simulink model "Model_TranslationEngine64"  (R2022b)
settings: Solver=FixedStepDiscrete  StartTime=0.0  StopTime=5  RelTol=1e-3  EnableMultiTasking=on
InitFcn:
  | % Initialize model
  | ModelSettings=BTConfig.GetModelSettings();
  | 
  | ModelSettings.Validate();
  | 
  | ModelInit;
  | 
  | 
  | % load library data
  | GainLibrary_data;
  | % Load saved values from partition process
  | CapturedConstMask.LoadMapFromFile(bdroot)
StartFcn:
  | % make sure all the simulated RTC requests are found
  | %RTC_SIM_OBJ.ValidateREQs();
undefined symbols (not defined in the file or in its folder): AA, BPLP, Column, NumHFRefBPF, NumHFRefLPF, NumMusicChannels, Row, VolumeMuteConfig
libraries: TuneVar x925, TOP x490, FeaturePath x111, CapturedConstLib x52
(part 20 of 34)

== system Model_TranslationEngine64/ModelPreAmp/DecRate/Medusa5H1/SleepingBeauty/SleepingBeauty/Enabled/MuteControl ==
  MuteControl : Subsystem  mask(Blocklib MuteControl){Config=InnerLinkConfig, FeatureName=MuteControl}
      mask prompts: Config "MuteControlConfig"; FeatureName "Mask feature name:"
      mask help: This component is to be used in conjunction with 1 or more instances of the MuteRamper block. There is no mask for this component. It provides the control layer for Mute processing via an RTC and tune variable, muteControlRampTime.
      mask init: same as Model_TranslationEngine64/PostProcess/PostProcess/Mute/Mute/MuteControl
      mask Help: If this control block is being used in a "multi-instance" manner, i.e. it is contorlling two or more MuteRamper blocks, there is an additional step that must be done. The developer must add a function-triggered subsytem containing an AND logic gate, which will combine the notification completion signals of the multiple ramper instances. The output of this subsytem must then feed the NTF_done input of the MuteControl block.
      mask Callback Config: BTConfig.CallbackHideIfPresent(gcbh,{'FeatureName'});
      mask TypeOptions FeatureName: FeaturePath/FeatureName

== system Model_TranslationEngine64/ModelPreAmp/DecRate/Medusa5H1/SleepingBeauty/SleepingBeauty/Enabled/SleepingBeautyDR ==
  InnerLink : Subsystem  mask(Blocklib SleepingBeauty){Config=InnerLinkConfig, FeatureName=SleepingBeautyDR}
      mask prompts: Config "SleepingBeautyConfig"; FeatureName "Feature path name:"
      mask help:
      | This block is to be used in conjunction with the Balance block.
      |
      | For the Channel to Ramper Map, enter any of the following values:
      | 1 - left channel
      | 2 - right channel
      | 3 - center channel
      | 4 - mono channel
      | -1 - unused channel (will esentially be muted)
      | (For headrest speakers, choose a seat-centric ramper, i.e. Left Seat Left Ear and Left Seat Right Ear would both be considered "Left content", receiving a 1).
      |
      | Silent Extreme Mutes Bass: Check this box if the intention is for mono channels to be muted upon Silent Extreme
      |
      | If this block is being used in a multi-instance application, be sure to give independent names in each instance's mask.
      mask init:
      | blkh=gcbh;
      | Config=BTConfig.Assert(blkh,Config);
      | 
      | SleepingBeautyMask.Init(blkh);
      | 
      | % Set boundary conditions
      | rampRateBounds = [5,50000];
      | rampTimeBounds = [1,3000];
      | 
      | BTConfig.InitSetFeatureIfPresent(blkh,'FeatureName');
      | Config.Validate();
      mask Callback Config: BTConfig.CallbackHideIfPresent(gcbh,{'FeatureName'});
      mask TypeOptions FeatureName: FeaturePath/FeatureName

== system Model_TranslationEngine64/ModelPreAmp/DecRate/Medusa5H1/SleepingBeauty/SleepingBeauty/Enabled/SleepingBeautyFR ==
  InnerLink : Subsystem  mask(Blocklib SleepingBeauty){Config=InnerLinkConfig, FeatureName=SleepingBeautyFR}
      mask prompts: Config "SleepingBeautyConfig"; FeatureName "Feature path name:"
      mask help:
      | This block is to be used in conjunction with the Balance block.
      |
      | For the Channel to Ramper Map, enter any of the following values:
      | 1 - left channel
      | 2 - right channel
      | 3 - center channel
      | 4 - mono channel
      | -1 - unused channel (will esentially be muted)
      | (For headrest speakers, choose a seat-centric ramper, i.e. Left Seat Left Ear and Left Seat Right Ear would both be considered "Left content", receiving a 1).
      |
      | Silent Extreme Mutes Bass: Check this box if the intention is for mono channels to be muted upon Silent Extreme
      |
      | If this block is being used in a multi-instance application, be sure to give independent names in each instance's mask.
      mask init: same as Model_TranslationEngine64/ModelPreAmp/DecRate/Medusa5H1/SleepingBeauty/SleepingBeauty/Enabled/SleepingBeautyDR/InnerLink
      mask Callback Config: BTConfig.CallbackHideIfPresent(gcbh,{'FeatureName'});
      mask TypeOptions FeatureName: FeaturePath/FeatureName

== system Model_TranslationEngine64/ModelPreAmp/DecRate/Medusa5H1/VLS/Crosstalk Cancellation/Pooliir with Non-Trivial Translations/InnerLink ==
  PoolIirTunableWithReset : Subsystem  mask(Bose Pool IIR Tunable){FeatureName=IIR, Config=Config}
      mask prompts: FeatureName "Filter name/purpose"; Config "PoolIirTunableWithResetConfig"
      mask help:
      | Pool IIR Tunable is a configurable multi-channel IIR filter that supports one or more channels. This block offers flexibility of tuning the number of stages and coefficients. Different filter coefficients and number of stages (biquads) can be used for each channel filter. The Pool IIR Tunable block supports different implementations, which could be configured at build-time:
      |
      | (i)   Generic: IIR filter code not optimized for any processor
      | (ii)  SharcCore: IIR filters executing on core (uses pooliir.asm CRL)
      | (iii) SharcGulAccel: IIR filters executing on IIR hardware accelerator, offloading MIPS usage from core
      | (iv) SharcGxpAccel: IIR filters take advantage of additional accelerators available on GXP processor
      | (v)  Hexagon: TBD
      |
      | NOTE: When using Pool IIR for Sharc-plus based processors, the codeWorkMemory buffer and input buffer should always be mapped to L1 memory to optimize MIPS utilization and avoid audio artifacts.
      |
      | For more information, please see 'Help'.
      mask init:
      | blkh=gcbh;
      | Config=BTConfig.Assert(blkh,Config);
      | 
      | BTConfig.InitSetFeatureIfPresent(blkh,'FeatureName');
      | Config.Validate();
      | Config.DoMaskInit(blkh);
      mask Help:
      | <b>Input signals: </b>
      | AudioIn: input channels [frame size x number of channels]
      | ResetTrigger: trigger to reset internal state buffer (usually preferred as a post RMDL step)
      | 
      | <b>Output signals: </b>
      | AudioOut: output channels [frame size x number of channels]
      | 
      | <b>Mask parameters: </b>
      | PoolIirTunableWithResetConfig
      | Filter name/purpose
      mask TypeOptions FeatureName: FeaturePath/FeatureName
      mask Callback Config: BTConfig.CallbackHideIfPresent(gcbh,{'FeatureName'});
      mask Display: DrawPoolIirIcon;

== system Model_TranslationEngine64/ModelPreAmp/PreAmpPart1/NEARPreAmp/Monoizer/Monoizer/MonoizerStereo/MonoizerCalc ==
  TuneTOP1 : Subsystem  mask(Talaria Trivial Tune TOP){TriggerInit=[385 412 535 498], TopName=G, TuneName=G, DataTypeOut=single, MaskValue=Config.G, TunabilityNumber=1, MinValue=[], MaxValue=[], BankNumber=0, PreOverlay=false, PostOverlay=false, UseSameName=on}
      mask prompts: TriggerInit "Hidden: MoveFcn redraw"; TopName "Name:"; TuneName "Name of TuneVar:"; DataTypeOut "Data type:"; MaskValue "Default Value:"; TunabilityNumber "Tunability:"; MinValue "Min Value:"; MaxValue "Max Value:"; BankNumber "Target memory bank number:"; PreOverlay "Requires pre-overlay action:"; PostOverlay "Requires post-overlay action:"; UseSameName "Use same name for tune variable and TOP"
      mask help: The TuneTOP block encapsultes a Target Overlay Parameter, a Tune Variable, and a Trivial Translation between them.
      mask init:
      | [ok,activeTopPath,activeTunePath] = TuneTOP_Mask.Init(gcbh);
      settings: MoveFcn=TuneTOP_Mask.CB_TriggerInit(gcbh);
      mask Callback TriggerInit: TuneTOP_Mask.CB_TriggerInit(gcbh);
      mask TypeOptions TopName: TOP/TopName
      mask TypeOptions TuneName: Tune Variable/TuneName
      mask TypeOptions DataTypeOut: TOP/DataTypeOut
      mask TypeOptions MaskValue: Tune Variable/MaskValue
      mask TypeOptions TunabilityNumber: Tune Variable/TunabilityNumber
      mask Callback TunabilityNumber: TuneVarMask.CB_TunabilityNumber(gcbh);
      mask TypeOptions MinValue: Tune Variable/MinValue
      mask TypeOptions MaxValue: Tune Variable/MaxValue
      mask TypeOptions BankNumber: TOP/BankNumber
      mask TypeOptions PreOverlay: TOP/PreOverlay
      mask TypeOptions PostOverlay: TOP/PostOverlay
      mask Callback UseSameName: TuneTOP_Mask.CB_UseSameName(gcbh);
      mask DialogControl toolPanel Prompt: Tuning Tool Hints
      mask DialogControl DescriptionGroup Prompt: Description
      mask DialogControl EditDescription Prompt: Edit Description
      mask DialogControl EditDescription Callback: TuneTOP_Mask.CB_EditDescription(gcbh);
      mask DialogControl TunabilityText Prompt: Easy: Changes nearly every tuning.
      mask DialogControl AdvancedPanel Prompt: Advanced
      mask DialogControl ConvertToFullTranslation Prompt: Irreversible conversion to full translation
      mask DialogControl ConvertToFullTranslation Callback: TuneTOP_Mask.CB_ConvertToFullTranslation(gcbh);
      mask DialogControl ErrorContainer Prompt: Error Messages
      mask Display:
      | % retrieve icon definition
      | [path,w,h] = TuneTOP_Mask.Icon();
      | 
      | % retrieve the block's pixel size
      | pos = get(gcbh,'position');
      | bw = pos(3) - pos(1);
      | bh = pos(4) - pos(2);
      | 
      | % draw centered icon
      | xAdj = bw/2 - w/2 + 5;
      | yAdj = bh/2 - h/2 + 4;
      | for i=1:length(path)
      | 	patch(path(i).x+xAdj, path(i).y+yAdj, path(i).rgb);
      | end
      | 
      | % show the top name or an X
      | if (exist('ok','var') && ok)
      | 	text(bw*0.5, bh*0.2, activeTopPath, 'horizontalAlignment', 'center');
      | 	patch(0,0,[1 1 1]);
      | 	patch(bw,bh,[1 1 1]);
      | else
      | 	tx=bw*0.03;
      | 	ty=bh*0.03;
      | 	patch([0 tx bw bw-tx], [ty 0 bh-ty bh], [1 0 0]);
      | 	patch([0 bw-tx bw tx], [bh-ty 0 ty bh], [1 0 0]);
      | end

== system Model_TranslationEngine64/NEAR/Near1p1/FrProc/Subsystem/FsEQFr/Pooliir/PoolIirTunableWithReset ==
  CapturedTuneConst : CapturedConstLib/CapturedConst  TriggerInit=[-600 302 -500 338]  Role=Automatic
      settings: SourceProductName=Bose Talaria
  FeaturePath : FeaturePath/FeaturePath  FeatureName=Pooliir  IsGroup=off  GroupNumber=-1  IsModule=off  TriggerInit=[-750 -81 -635 26]
      settings: SourceProductName=Bose Talaria
  TOP : TOP/TOP  TriggerInit=[-145 187 5 243]  TopName=PooliirNumStages  DataTypeOut=uint32  BankNumber=0  PreOverlay=false  PostOverlay=Config.VariantObj.PostOverlayRequired  Role=Automatic
      settings: SourceProductName=Bose Talaria
  TOP1 : TOP/TOP  TriggerInit=[-140 277 10 333]  TopName=pooliirCoeffs  DataTypeOut=single  BankNumber=0  PreOverlay=false  PostOverlay=Config.VariantObj.PostOverlayRequired  Role=Automatic
      settings: SourceProductName=Bose Talaria
  TranslateTrigger : TuneVar/TranslateTrigger  TriggerInit=[-339 35 -301 90]
      settings: SourceProductName=Bose Talaria
  Translation : MATLAB Function  TreatAsAtomicUnit=on  mask{MaxNumStages=Config.MaxNumStages, VariantUint8=Config.Variant.Uint8Str}
      mask prompts: VariantUint8 "Variant"
  Tune Variable1 : TuneVar/TuneVar  TuneName=numStages  SpecifyMaxSize=off  VariableDim=1 (Row)  MaxSize=[1 1]  TunabilityNumber=1  MinValue=[]  MaxValue=[]  TriggerInit=[-750 235 -580 285]  MaskValue=Config.TuneDefaults.NumStages
      settings: SourceProductName=Bose Talaria
  Tune Variable2 : TuneVar/TuneVar  TuneName=sosCoefficients  SpecifyMaxSize=on  VariableDim=1 (Row)  MaxSize=[Config.MaxNumStages 6]  TunabilityNumber=1  MinValue=[]  MaxValue=[]  TriggerInit=[-750 175 -580 225]  MaskValue=Config.TuneDefaults.SosCoefficients
      settings: SourceProductName=Bose Talaria
  wires:
  TranslateTrigger/1 -> Translation/Trigger
  Tune Variable2/1 -> Translation/1(RawSOS)  "sosCoefficients"
  Translation/2(PoolCoeffs) -> TOP1/1
  Translation/1(PoolNumStages) -> TOP/1
  Tune Variable1/1 -> Translation/2(NumStages)  "numStages"
  CapturedTuneConst/1 -> Translation/3(NumChannels)

== system Model_TranslationEngine64/NEAR/Near1p1/FrProc/Subsystem/FsEQFr/Subsystem1/Subsystem ==
  Tune Variable : TuneVar/TuneVar  TuneName=f1_del  SpecifyMaxSize=off  VariableDim=1 (Row)  MaxSize=[1 1]  TunabilityNumber=1  MinValue=[]  MaxValue=[]  TriggerInit=[20 20 190 70]  MaskValue=Config.f1_del
      settings: SourceProductName=Bose Talaria
  Tune Variable1 : TuneVar/TuneVar  TuneName=f2_del  SpecifyMaxSize=off  VariableDim=1 (Row)  MaxSize=[1 1]  TunabilityNumber=1  MinValue=[]  MaxValue=[]  TriggerInit=[20 155 190 205]  MaskValue=Config.f2_del
      settings: SourceProductName=Bose Talaria
  Tune Variable2 : TuneVar/TuneVar  TuneName=f3_del  SpecifyMaxSize=off  VariableDim=1 (Row)  MaxSize=[1 1]  TunabilityNumber=1  MinValue=[]  MaxValue=[]  TriggerInit=[20 290 190 340]  MaskValue=Config.f3_del
      settings: SourceProductName=Bose Talaria
  Tune Variable3 : TuneVar/TuneVar  TuneName=f4_del  SpecifyMaxSize=off  VariableDim=1 (Row)  MaxSize=[1 1]  TunabilityNumber=1  MinValue=[]  MaxValue=[]  TriggerInit=[20 425 190 475]  MaskValue=Config.f4_del
      settings: SourceProductName=Bose Talaria
  Tune Variable4 : TuneVar/TuneVar  TuneName=f5_del  SpecifyMaxSize=off  VariableDim=1 (Row)  MaxSize=[1 1]  TunabilityNumber=1  MinValue=[]  MaxValue=[]  TriggerInit=[20 560 190 610]  MaskValue=Config.f5_del
      settings: SourceProductName=Bose Talaria
  Tune Variable5 : TuneVar/TuneVar  TuneName=f6_del  SpecifyMaxSize=off  VariableDim=1 (Row)  MaxSize=[1 1]  TunabilityNumber=1  MinValue=[]  MaxValue=[]  TriggerInit=[20 695 190 745]  MaskValue=Config.f6_del
      settings: SourceProductName=Bose Talaria
  Tune Variable7 : TuneVar/TuneVar  TuneName=f7_del  SpecifyMaxSize=off  VariableDim=1 (Row)  MaxSize=[1 1]  TunabilityNumber=1  MinValue=[]  MaxValue=[]  TriggerInit=[20 825 190 875]  MaskValue=Config.f7_del
      settings: SourceProductName=Bose Talaria
  f1 : Outport
  f2 : Outport  Port=2
  f3 : Outport  Port=3
  f4 : Outport  Port=4
  f5 : Outport  Port=5
  f6 : Outport  Port=6
  f7 : Outport  Port=7
  wires:
  Tune Variable5/1 -> f6/1  "f6_del"
  Tune Variable2/1 -> f3/1  "f3_del"
  Tune Variable7/1 -> f7/1  "f7_del"
  Tune Variable/1 -> f1/1  "f1_del"
  Tune Variable1/1 -> f2/1  "f2_del"
  Tune Variable3/1 -> f4/1  "f4_del"
  Tune Variable4/1 -> f5/1  "f5_del"

== system Model_TranslationEngine64/NEAR/Near1p1/FrProc/Subsystem/HrEQFr/PoolIirTunable/PoolIirTunableWithReset ==
  CapturedTuneConst : CapturedConstLib/CapturedConst  TriggerInit=[-600 302 -500 338]  Role=Automatic
      settings: SourceProductName=Bose Talaria
  FeaturePath : FeaturePath/FeaturePath  FeatureName=PoolIirTunable  IsGroup=off  GroupNumber=-1  IsModule=off  TriggerInit=[-750 -81 -635 26]
      settings: SourceProductName=Bose Talaria
  TOP : TOP/TOP  TriggerInit=[-145 187 5 243]  TopName=PooliirNumStages  DataTypeOut=uint32  BankNumber=0  PreOverlay=false  PostOverlay=Config.VariantObj.PostOverlayRequired  Role=Automatic
      settings: SourceProductName=Bose Talaria
  TOP1 : TOP/TOP  TriggerInit=[-140 277 10 333]  TopName=pooliirCoeffs  DataTypeOut=single  BankNumber=0  PreOverlay=false  PostOverlay=Config.VariantObj.PostOverlayRequired  Role=Automatic
      settings: SourceProductName=Bose Talaria
  TranslateTrigger : TuneVar/TranslateTrigger  TriggerInit=[-339 35 -301 90]
      settings: SourceProductName=Bose Talaria
  Translation : MATLAB Function  TreatAsAtomicUnit=on  mask{MaxNumStages=Config.MaxNumStages, VariantUint8=Config.Variant.Uint8Str}
      mask prompts: VariantUint8 "Variant"
  Tune Variable1 : TuneVar/TuneVar  TuneName=numStages  SpecifyMaxSize=off  VariableDim=1 (Row)  MaxSize=[1 1]  TunabilityNumber=1  MinValue=[]  MaxValue=[]  TriggerInit=[-750 235 -580 285]  MaskValue=Config.TuneDefaults.NumStages
      settings: SourceProductName=Bose Talaria
  Tune Variable2 : TuneVar/TuneVar  TuneName=sosCoefficients  SpecifyMaxSize=on  VariableDim=1 (Row)  MaxSize=[Config.MaxNumStages 6]  TunabilityNumber=1  MinValue=[]  MaxValue=[]  TriggerInit=[-750 175 -580 225]  MaskValue=Config.TuneDefaults.SosCoefficients
      settings: SourceProductName=Bose Talaria
  wires:
  TranslateTrigger/1 -> Translation/Trigger
  Tune Variable2/1 -> Translation/1(RawSOS)  "sosCoefficients"
  Translation/2(PoolCoeffs) -> TOP1/1
  Translation/1(PoolNumStages) -> TOP/1
  Tune Variable1/1 -> Translation/2(NumStages)  "numStages"
  CapturedTuneConst/1 -> Translation/3(NumChannels)

== system Model_TranslationEngine64/NEAR/Near1p1/FrProc/Subsystem/HrEQFr/Subsystem2/Subsystem ==
  Tune Variable1 : TuneVar/TuneVar  TuneName=driver_src1  SpecifyMaxSize=off  VariableDim=1 (Row)  MaxSize=[1 1]  TunabilityNumber=1  MinValue=[]  MaxValue=[]  TriggerInit=[35 385 205 435]  MaskValue=Config.driver_src1
      settings: SourceProductName=Bose Talaria
  Tune Variable2 : TuneVar/TuneVar  TuneName=driver_src2  SpecifyMaxSize=off  VariableDim=1 (Row)  MaxSize=[1 1]  TunabilityNumber=1  MinValue=[]  MaxValue=[]  TriggerInit=[35 515 205 565]  MaskValue=Config.driver_src2
      settings: SourceProductName=Bose Talaria
  Tune Variable3 : TuneVar/TuneVar  TuneName=driver_src3  SpecifyMaxSize=off  VariableDim=1 (Row)  MaxSize=[1 1]  TunabilityNumber=1  MinValue=[]  MaxValue=[]  TriggerInit=[35 620 205 670]  MaskValue=Config.driver_src3
      settings: SourceProductName=Bose Talaria
  Tune Variable4 : TuneVar/TuneVar  TuneName=driver_src4  SpecifyMaxSize=off  VariableDim=1 (Row)  MaxSize=[1 1]  TunabilityNumber=1  MinValue=[]  MaxValue=[]  TriggerInit=[35 750 205 800]  MaskValue=Config.driver_src4
      settings: SourceProductName=Bose Talaria
  Tune Variable5 : TuneVar/TuneVar  TuneName=passenger_src1  SpecifyMaxSize=off  VariableDim=1 (Row)  MaxSize=[1 1]  TunabilityNumber=1  MinValue=[]  MaxValue=[]  TriggerInit=[35 880 205 930]  MaskValue=Config.passenger_src1
      settings: SourceProductName=Bose Talaria
  Tune Variable6 : TuneVar/TuneVar  TuneName=passenger_src3  SpecifyMaxSize=off  VariableDim=1 (Row)  MaxSize=[1 1]  TunabilityNumber=1  MinValue=[]  MaxValue=[]  TriggerInit=[35 1140 205 1190]  MaskValue=Config.passenger_src3
      settings: SourceProductName=Bose Talaria
  Tune Variable7 : TuneVar/TuneVar  TuneName=passenger_src2  SpecifyMaxSize=off  VariableDim=1 (Row)  MaxSize=[1 1]  TunabilityNumber=1  MinValue=[]  MaxValue=[]  TriggerInit=[35 1010 205 1060]  MaskValue=Config.passenger_src2
      settings: SourceProductName=Bose Talaria
  Tune Variable8 : TuneVar/TuneVar  TuneName=passenger_src4  SpecifyMaxSize=off  VariableDim=1 (Row)  MaxSize=[1 1]  TunabilityNumber=1  MinValue=[]  MaxValue=[]  TriggerInit=[30 1285 200 1335]  MaskValue=Config.passenger_src4
      settings: SourceProductName=Bose Talaria
  driver_src1 : Outport
  driver_src2 : Outport  Port=2
  driver_src3 : Outport  Port=3
  driver_src4 : Outport  Port=4
  passenger_src1 : Outport  Port=5
  passenger_src2 : Outport  Port=6
  passenger_src3 : Outport  Port=7
  passenger_src4 : Outport  Port=8
  wires:
  Tune Variable5/1 -> passenger_src1/1  "passenger_src1"
  Tune Variable7/1 -> passenger_src2/1  "passenger_src2"
  Tune Variable8/1 -> passenger_src4/1  "passenger_src4"
  Tune Variable6/1 -> passenger_src3/1  "passenger_src3"
  Tune Variable4/1 -> driver_src4/1  "driver_src4"
  Tune Variable3/1 -> driver_src3/1  "driver_src3"
  Tune Variable2/1 -> driver_src2/1  "driver_src2"
  Tune Variable1/1 -> driver_src1/1  "driver_src1"

== system Model_TranslationEngine64/NEAR/Near1p1/FrProc/Subsystem/Upmixer1p1Fr/Subsystem1/Subsystem ==
  Tune Variable : TuneVar/TuneVar  TuneName=f1_mix  SpecifyMaxSize=off  VariableDim=1 (Row)  MaxSize=[1 1]  TunabilityNumber=1  MinValue=[]  MaxValue=[]  TriggerInit=[20 20 190 70]  MaskValue=Config.TuneDefaults.f1_mix
      settings: SourceProductName=Bose Talaria
  Tune Variable1 : TuneVar/TuneVar  TuneName=f2_mix  SpecifyMaxSize=off  VariableDim=1 (Row)  MaxSize=[1 1]  TunabilityNumber=1  MinValue=[]  MaxValue=[]  TriggerInit=[20 155 190 205]  MaskValue=Config.TuneDefaults.f2_mix
      settings: SourceProductName=Bose Talaria
  Tune Variable2 : TuneVar/TuneVar  TuneName=f3_mix  SpecifyMaxSize=off  VariableDim=1 (Row)  MaxSize=[1 1]  TunabilityNumber=1  MinValue=[]  MaxValue=[]  TriggerInit=[20 290 190 340]  MaskValue=Config.TuneDefaults.f3_mix
      settings: SourceProductName=Bose Talaria
  Tune Variable3 : TuneVar/TuneVar  TuneName=f4_mix  SpecifyMaxSize=off  VariableDim=1 (Row)  MaxSize=[1 1]  TunabilityNumber=1  MinValue=[]  MaxValue=[]  TriggerInit=[20 425 190 475]  MaskValue=Config.TuneDefaults.f4_mix
      settings: SourceProductName=Bose Talaria
  Tune Variable4 : TuneVar/TuneVar  TuneName=f5_mix  SpecifyMaxSize=off  VariableDim=1 (Row)  MaxSize=[1 1]  TunabilityNumber=1  MinValue=[]  MaxValue=[]  TriggerInit=[20 560 190 610]  MaskValue=Config.TuneDefaults.f5_mix
      settings: SourceProductName=Bose Talaria
  Tune Variable5 : TuneVar/TuneVar  TuneName=f6_mix  SpecifyMaxSize=off  VariableDim=1 (Row)  MaxSize=[1 1]  TunabilityNumber=1  MinValue=[]  MaxValue=[]  TriggerInit=[20 695 190 745]  MaskValue=Config.TuneDefaults.f6_mix
      settings: SourceProductName=Bose Talaria
  Tune Variable7 : TuneVar/TuneVar  TuneName=f7_mix  SpecifyMaxSize=off  VariableDim=1 (Row)  MaxSize=[1 1]  TunabilityNumber=1  MinValue=[]  MaxValue=[]  TriggerInit=[20 825 190 875]  MaskValue=Config.TuneDefaults.f7_mix
      settings: SourceProductName=Bose Talaria
  f1 : Outport
  f2 : Outport  Port=2
  f3 : Outport  Port=3
  f4 : Outport  Port=4
  f5 : Outport  Port=5
  f6 : Outport  Port=6
  f7 : Outport  Port=7
  wires:
  Tune Variable5/1 -> f6/1  "f6_mix"
  Tune Variable2/1 -> f3/1  "f3_mix"
  Tune Variable7/1 -> f7/1  "f7_mix"
  Tune Variable/1 -> f1/1  "f1_mix"
  Tune Variable1/1 -> f2/1  "f2_mix"
  Tune Variable3/1 -> f4/1  "f4_mix"
  Tune Variable4/1 -> f5/1  "f5_mix"

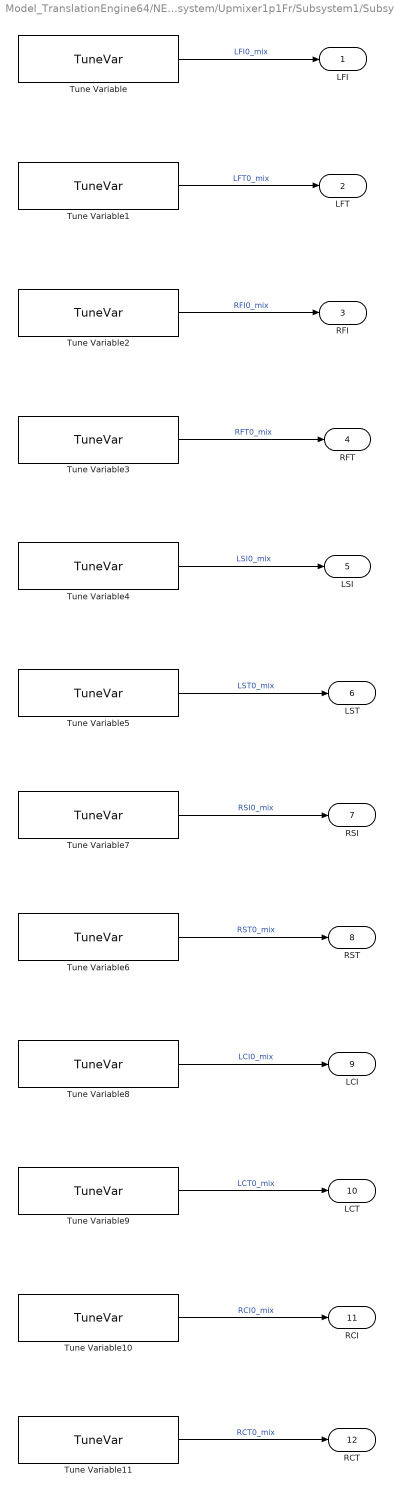
== system Model_TranslationEngine64/NEAR/Near1p1/FrProc/Subsystem/Upmixer1p1Fr/Subsystem1/Subsystem1 ==
  Tune Variable : TuneVar/TuneVar  TuneName=LFI0_mix  SpecifyMaxSize=off  VariableDim=1 (Row)  MaxSize=[1 1]  TunabilityNumber=1  MinValue=[]  MaxValue=[]  TriggerInit=[1315 -1070 1485 -1020]  MaskValue=Config.TuneDefaults.LFI0_mix
      settings: SourceProductName=Bose Talaria
  Tune Variable1 : TuneVar/TuneVar  TuneName=LFT0_mix  SpecifyMaxSize=off  VariableDim=1 (Row)  MaxSize=[1 1]  TunabilityNumber=1  MinValue=[]  MaxValue=[]  TriggerInit=[1315 -935 1485 -885]  MaskValue=Config.TuneDefaults.LFT0_mix
      settings: SourceProductName=Bose Talaria
  Tune Variable10 : TuneVar/TuneVar  TuneName=RCI0_mix  SpecifyMaxSize=off  VariableDim=1 (Row)  MaxSize=[1 1]  TunabilityNumber=1  MinValue=[]  MaxValue=[]  TriggerInit=[1315 270 1485 320]  MaskValue=Config.TuneDefaults.RCI0_mix
      settings: SourceProductName=Bose Talaria
  Tune Variable11 : TuneVar/TuneVar  TuneName=RCT0_mix  SpecifyMaxSize=off  VariableDim=1 (Row)  MaxSize=[1 1]  TunabilityNumber=1  MinValue=[]  MaxValue=[]  TriggerInit=[1315 400 1485 450]  MaskValue=Config.TuneDefaults.RCT0_mix
      settings: SourceProductName=Bose Talaria
  Tune Variable2 : TuneVar/TuneVar  TuneName=RFI0_mix  SpecifyMaxSize=off  VariableDim=1 (Row)  MaxSize=[1 1]  TunabilityNumber=1  MinValue=[]  MaxValue=[]  TriggerInit=[1315 -800 1485 -750]  MaskValue=Config.TuneDefaults.RFI0_mix
      settings: SourceProductName=Bose Talaria
  Tune Variable3 : TuneVar/TuneVar  TuneName=RFT0_mix  SpecifyMaxSize=off  VariableDim=1 (Row)  MaxSize=[1 1]  TunabilityNumber=1  MinValue=[]  MaxValue=[]  TriggerInit=[1315 -665 1485 -615]  MaskValue=Config.TuneDefaults.RFT0_mix
      settings: SourceProductName=Bose Talaria
  Tune Variable4 : TuneVar/TuneVar  TuneName=LSI0_mix  SpecifyMaxSize=off  VariableDim=1 (Row)  MaxSize=[1 1]  TunabilityNumber=1  MinValue=[]  MaxValue=[]  TriggerInit=[1315 -530 1485 -480]  MaskValue=Config.TuneDefaults.LSI0_mix
      settings: SourceProductName=Bose Talaria
  Tune Variable5 : TuneVar/TuneVar  TuneName=LST0_mix  SpecifyMaxSize=off  VariableDim=1 (Row)  MaxSize=[1 1]  TunabilityNumber=1  MinValue=[]  MaxValue=[]  TriggerInit=[1315 -395 1485 -345]  MaskValue=Config.TuneDefaults.LST0_mix
      settings: SourceProductName=Bose Talaria
  Tune Variable6 : TuneVar/TuneVar  TuneName=RST0_mix  SpecifyMaxSize=off  VariableDim=1 (Row)  MaxSize=[1 1]  TunabilityNumber=1  MinValue=[]  MaxValue=[]  TriggerInit=[1315 -135 1485 -85]  MaskValue=Config.TuneDefaults.RST0_mix
      settings: SourceProductName=Bose Talaria
  Tune Variable7 : TuneVar/TuneVar  TuneName=RSI0_mix  SpecifyMaxSize=off  VariableDim=1 (Row)  MaxSize=[1 1]  TunabilityNumber=1  MinValue=[]  MaxValue=[]  TriggerInit=[1315 -265 1485 -215]  MaskValue=Config.TuneDefaults.RSI0_mix
      settings: SourceProductName=Bose Talaria
  Tune Variable8 : TuneVar/TuneVar  TuneName=LCI0_mix  SpecifyMaxSize=off  VariableDim=1 (Row)  MaxSize=[1 1]  TunabilityNumber=1  MinValue=[]  MaxValue=[]  TriggerInit=[20 1090 190 1140]  MaskValue=Config.TuneDefaults.LCI0_mix
      settings: SourceProductName=Bose Talaria
  Tune Variable9 : TuneVar/TuneVar  TuneName=LCT0_mix  SpecifyMaxSize=off  VariableDim=1 (Row)  MaxSize=[1 1]  TunabilityNumber=1  MinValue=[]  MaxValue=[]  TriggerInit=[1315 135 1485 185]  MaskValue=Config.TuneDefaults.LCT0_mix
      settings: SourceProductName=Bose Talaria
  LFI : Outport
  LFT : Outport  Port=2
  RFI : Outport  Port=3
  RFT : Outport  Port=4
  LSI : Outport  Port=5
  LST : Outport  Port=6
  RSI : Outport  Port=7
  RST : Outport  Port=8
  LCI : Outport  Port=9
  LCT : Outport  Port=10
  RCI : Outport  Port=11
  RCT : Outport  Port=12
  wires:
  Tune Variable1/1 -> LFT/1  "LFT0_mix"
  Tune Variable11/1 -> RCT/1  "RCT0_mix"
  Tune Variable6/1 -> RST/1  "RST0_mix"
  Tune Variable3/1 -> RFT/1  "RFT0_mix"
  Tune Variable/1 -> LFI/1  "LFI0_mix"
  Tune Variable2/1 -> RFI/1  "RFI0_mix"
  Tune Variable7/1 -> RSI/1  "RSI0_mix"
  Tune Variable4/1 -> LSI/1  "LSI0_mix"
  Tune Variable8/1 -> LCI/1  "LCI0_mix"
  Tune Variable5/1 -> LST/1  "LST0_mix"
  Tune Variable9/1 -> LCT/1  "LCT0_mix"
  Tune Variable10/1 -> RCI/1  "RCI0_mix"

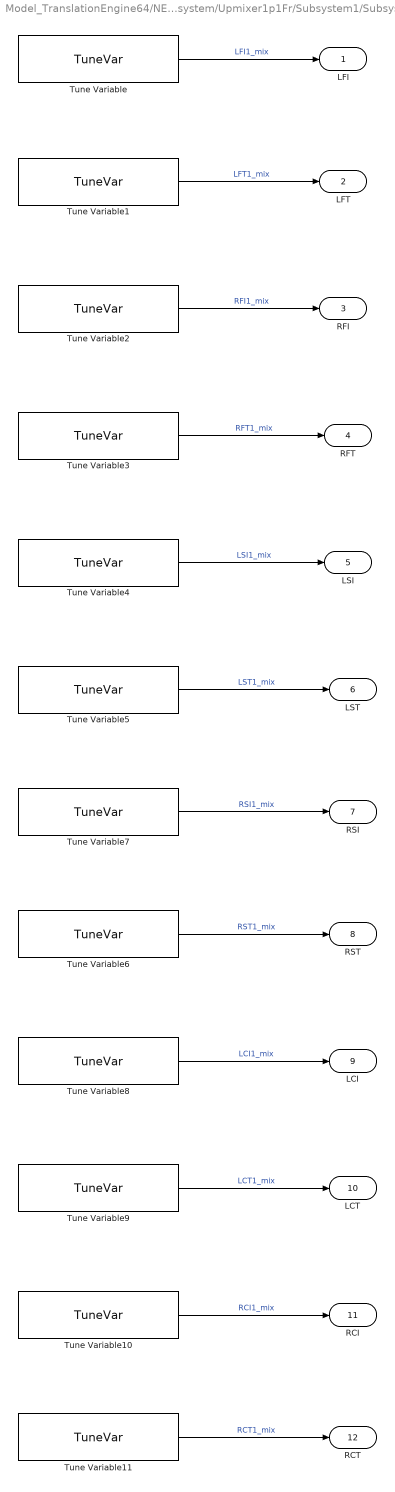
== system Model_TranslationEngine64/NEAR/Near1p1/FrProc/Subsystem/Upmixer1p1Fr/Subsystem1/Subsystem2 ==
  Tune Variable : TuneVar/TuneVar  TuneName=LFI1_mix  SpecifyMaxSize=off  VariableDim=1 (Row)  MaxSize=[1 1]  TunabilityNumber=1  MinValue=[]  MaxValue=[]  TriggerInit=[1315 910 1485 960]  MaskValue=Config.TuneDefaults.LFI1_mix
      settings: SourceProductName=Bose Talaria
  Tune Variable1 : TuneVar/TuneVar  TuneName=LFT1_mix  SpecifyMaxSize=off  VariableDim=1 (Row)  MaxSize=[1 1]  TunabilityNumber=1  MinValue=[]  MaxValue=[]  TriggerInit=[1315 1040 1485 1090]  MaskValue=Config.TuneDefaults.LFT1_mix
      settings: SourceProductName=Bose Talaria
  Tune Variable10 : TuneVar/TuneVar  TuneName=RCI1_mix  SpecifyMaxSize=off  VariableDim=1 (Row)  MaxSize=[1 1]  TunabilityNumber=1  MinValue=[]  MaxValue=[]  TriggerInit=[1315 2245 1485 2295]  MaskValue=Config.TuneDefaults.RCI1_mix
      settings: SourceProductName=Bose Talaria
  Tune Variable11 : TuneVar/TuneVar  TuneName=RCT1_mix  SpecifyMaxSize=off  VariableDim=1 (Row)  MaxSize=[1 1]  TunabilityNumber=1  MinValue=[]  MaxValue=[]  TriggerInit=[1315 2375 1485 2425]  MaskValue=Config.TuneDefaults.RCT1_mix
      settings: SourceProductName=Bose Talaria
  Tune Variable2 : TuneVar/TuneVar  TuneName=RFI1_mix  SpecifyMaxSize=off  VariableDim=1 (Row)  MaxSize=[1 1]  TunabilityNumber=1  MinValue=[]  MaxValue=[]  TriggerInit=[1315 1175 1485 1225]  MaskValue=Config.TuneDefaults.RFI1_mix
      settings: SourceProductName=Bose Talaria
  Tune Variable3 : TuneVar/TuneVar  TuneName=RFT1_mix  SpecifyMaxSize=off  VariableDim=1 (Row)  MaxSize=[1 1]  TunabilityNumber=1  MinValue=[]  MaxValue=[]  TriggerInit=[1315 1310 1485 1360]  MaskValue=Config.TuneDefaults.RFT1_mix
      settings: SourceProductName=Bose Talaria
  Tune Variable4 : TuneVar/TuneVar  TuneName=LSI1_mix  SpecifyMaxSize=off  VariableDim=1 (Row)  MaxSize=[1 1]  TunabilityNumber=1  MinValue=[]  MaxValue=[]  TriggerInit=[1315 1445 1485 1495]  MaskValue=Config.TuneDefaults.LSI1_mix
      settings: SourceProductName=Bose Talaria
  Tune Variable5 : TuneVar/TuneVar  TuneName=LST1_mix  SpecifyMaxSize=off  VariableDim=1 (Row)  MaxSize=[1 1]  TunabilityNumber=1  MinValue=[]  MaxValue=[]  TriggerInit=[1315 1580 1485 1630]  MaskValue=Config.TuneDefaults.LST1_mix
      settings: SourceProductName=Bose Talaria
  Tune Variable6 : TuneVar/TuneVar  TuneName=RST1_mix  SpecifyMaxSize=off  VariableDim=1 (Row)  MaxSize=[1 1]  TunabilityNumber=1  MinValue=[]  MaxValue=[]  TriggerInit=[1315 1840 1485 1890]  MaskValue=Config.TuneDefaults.RST1_mix
      settings: SourceProductName=Bose Talaria
  Tune Variable7 : TuneVar/TuneVar  TuneName=RSI1_mix  SpecifyMaxSize=off  VariableDim=1 (Row)  MaxSize=[1 1]  TunabilityNumber=1  MinValue=[]  MaxValue=[]  TriggerInit=[1315 1710 1485 1760]  MaskValue=Config.TuneDefaults.RSI1_mix
      settings: SourceProductName=Bose Talaria
  Tune Variable8 : TuneVar/TuneVar  TuneName=LCI1_mix  SpecifyMaxSize=off  VariableDim=1 (Row)  MaxSize=[1 1]  TunabilityNumber=1  MinValue=[]  MaxValue=[]  TriggerInit=[1315 1975 1485 2025]  MaskValue=Config.TuneDefaults.LCI1_mix
      settings: SourceProductName=Bose Talaria
  Tune Variable9 : TuneVar/TuneVar  TuneName=LCT1_mix  SpecifyMaxSize=off  VariableDim=1 (Row)  MaxSize=[1 1]  TunabilityNumber=1  MinValue=[]  MaxValue=[]  TriggerInit=[1315 2110 1485 2160]  MaskValue=Config.TuneDefaults.LCT1_mix
      settings: SourceProductName=Bose Talaria
  LFI : Outport
  LFT : Outport  Port=2
  RFI : Outport  Port=3
  RFT : Outport  Port=4
  LSI : Outport  Port=5
  LST : Outport  Port=6
  RSI : Outport  Port=7
  RST : Outport  Port=8
  LCI : Outport  Port=9
  LCT : Outport  Port=10
  RCI : Outport  Port=11
  RCT : Outport  Port=12
  wires:
  Tune Variable3/1 -> RFT/1  "RFT1_mix"
  Tune Variable/1 -> LFI/1  "LFI1_mix"
  Tune Variable7/1 -> RSI/1  "RSI1_mix"
  Tune Variable2/1 -> RFI/1  "RFI1_mix"
  Tune Variable4/1 -> LSI/1  "LSI1_mix"
  Tune Variable1/1 -> LFT/1  "LFT1_mix"
  Tune Variable11/1 -> RCT/1  "RCT1_mix"
  Tune Variable5/1 -> LST/1  "LST1_mix"
  Tune Variable6/1 -> RST/1  "RST1_mix"
  Tune Variable8/1 -> LCI/1  "LCI1_mix"
  Tune Variable9/1 -> LCT/1  "LCT1_mix"
  Tune Variable10/1 -> RCI/1  "RCI1_mix"

== system Model_TranslationEngine64/NEAR/Near1p1/FrProc/Subsystem/Upmixer1p1Fr/Subsystem1/Subsystem3 ==
  Tune Variable : TuneVar/TuneVar  TuneName=nv0l_mix  SpecifyMaxSize=off  VariableDim=1 (Row)  MaxSize=[1 1]  TunabilityNumber=1  MinValue=[]  MaxValue=[]  TriggerInit=[1345 730 1515 780]  MaskValue=Config.TuneDefaults.nv0l_mix
      settings: SourceProductName=Bose Talaria
  Tune Variable1 : TuneVar/TuneVar  TuneName=nv0r_mix  SpecifyMaxSize=off  VariableDim=1 (Row)  MaxSize=[1 1]  TunabilityNumber=1  MinValue=[]  MaxValue=[]  TriggerInit=[1345 865 1515 915]  MaskValue=Config.TuneDefaults.nv0r_mix
      settings: SourceProductName=Bose Talaria
  Tune Variable2 : TuneVar/TuneVar  TuneName=nv1l_mix  SpecifyMaxSize=off  VariableDim=1 (Row)  MaxSize=[1 1]  TunabilityNumber=1  MinValue=[]  MaxValue=[]  TriggerInit=[1345 1000 1515 1050]  MaskValue=Config.TuneDefaults.nv1l_mix
      settings: SourceProductName=Bose Talaria
  Tune Variable3 : TuneVar/TuneVar  TuneName=nv1r_mix  SpecifyMaxSize=off  VariableDim=1 (Row)  MaxSize=[1 1]  TunabilityNumber=1  MinValue=[]  MaxValue=[]  TriggerInit=[1345 1135 1515 1185]  MaskValue=Config.TuneDefaults.nv1r_mix
      settings: SourceProductName=Bose Talaria
  nv0l : Outport
  nv0r : Outport  Port=2
  nv1l : Outport  Port=3
  nv1r : Outport  Port=4
  wires:
  Tune Variable1/1 -> nv0r/1  "nv0r_mix"
  Tune Variable/1 -> nv0l/1  "nv0l_mix"
  Tune Variable3/1 -> nv1r/1  "nv1r_mix"
  Tune Variable2/1 -> nv1l/1  "nv1l_mix"

== system Model_TranslationEngine64/NEAR/Near1p1/VolumeMute/AnnouncementLevelDetector/PreProcessing/PreEmphasisShelfFilter/PoolIirTunableWithReset ==
  CapturedTuneConst : CapturedConstLib/CapturedConst  TriggerInit=[-600 302 -500 338]  Role=Automatic
      settings: SourceProductName=Bose Talaria
  FeaturePath : FeaturePath/FeaturePath  FeatureName=PreEmphasisShelfFilter  IsGroup=off  GroupNumber=-1  IsModule=off  TriggerInit=[-750 -81 -635 26]
      settings: SourceProductName=Bose Talaria
  TOP : TOP/TOP  TriggerInit=[-145 187 5 243]  TopName=PooliirNumStages  DataTypeOut=uint32  BankNumber=0  PreOverlay=false  PostOverlay=Config.VariantObj.PostOverlayRequired  Role=Automatic
      settings: SourceProductName=Bose Talaria
  TOP1 : TOP/TOP  TriggerInit=[-140 277 10 333]  TopName=pooliirCoeffs  DataTypeOut=single  BankNumber=0  PreOverlay=false  PostOverlay=Config.VariantObj.PostOverlayRequired  Role=Automatic
      settings: SourceProductName=Bose Talaria
  TranslateTrigger : TuneVar/TranslateTrigger  TriggerInit=[-339 35 -301 90]
      settings: SourceProductName=Bose Talaria
  Translation : MATLAB Function  TreatAsAtomicUnit=on  mask{MaxNumStages=Config.MaxNumStages, VariantUint8=Config.Variant.Uint8Str}
      mask prompts: VariantUint8 "Variant"
  Tune Variable1 : TuneVar/TuneVar  TuneName=numStages  SpecifyMaxSize=off  VariableDim=1 (Row)  MaxSize=[1 1]  TunabilityNumber=1  MinValue=[]  MaxValue=[]  TriggerInit=[-750 235 -580 285]  MaskValue=Config.TuneDefaults.NumStages
      settings: SourceProductName=Bose Talaria
  Tune Variable2 : TuneVar/TuneVar  TuneName=sosCoefficients  SpecifyMaxSize=on  VariableDim=1 (Row)  MaxSize=[Config.MaxNumStages 6]  TunabilityNumber=1  MinValue=[]  MaxValue=[]  TriggerInit=[-750 175 -580 225]  MaskValue=Config.TuneDefaults.SosCoefficients
      settings: SourceProductName=Bose Talaria
  wires:
  TranslateTrigger/1 -> Translation/Trigger
  Tune Variable2/1 -> Translation/1(RawSOS)  "sosCoefficients"
  Translation/2(PoolCoeffs) -> TOP1/1
  Translation/1(PoolNumStages) -> TOP/1
  Tune Variable1/1 -> Translation/2(NumStages)  "numStages"
  CapturedTuneConst/1 -> Translation/3(NumChannels)

== system Model_TranslationEngine64/NEAR/Near1p1/VolumeMute/VolMuteCh1/Ann1NonEntGainCalc/vncSignal/TuneTOP ==
  TOP : TOP/TOP  TriggerInit=[440 20 585 80]  TopName=MinVncSignal  DataTypeOut=single  BankNumber=BankNumber  PreOverlay=PreOverlay  PostOverlay=PostOverlay  Role=Automatic
      settings: SourceProductName=Bose Talaria
  TrivialTranslation : TuneVar/TrivialTranslation  TriggerInit=[300 28 350 72]
      settings: SourceProductName=Bose Talaria
  Tune Variable : TuneVar/TuneVar  TuneName=MinVncSignal  SpecifyMaxSize=off  VariableDim=1 (Row)  MaxSize=[1 1]  TunabilityNumber=1  MinValue=MinValue  MaxValue=MaxValue  TriggerInit=[20 25 190 75]  MaskValue=MaskValue
      settings: SourceProductName=Bose Talaria
  wires:
  Tune Variable/1 -> TrivialTranslation/1  "MinVncSignal"
  TrivialTranslation/1 -> TOP/1

== system Model_TranslationEngine64/NEAR/Near1p1/VolumeMute/VolMuteCh1/Ann1NonEntGainCalc/vncSignal/TuneTOP1 ==
  TOP : TOP/TOP  TriggerInit=[440 20 585 80]  TopName=MaxSpl  DataTypeOut=single  BankNumber=BankNumber  PreOverlay=PreOverlay  PostOverlay=PostOverlay  Role=Automatic
      settings: SourceProductName=Bose Talaria
  TrivialTranslation : TuneVar/TrivialTranslation  TriggerInit=[300 28 350 72]
      settings: SourceProductName=Bose Talaria
  Tune Variable : TuneVar/TuneVar  TuneName=MaxSpl  SpecifyMaxSize=off  VariableDim=1 (Row)  MaxSize=[1 1]  TunabilityNumber=1  MinValue=MinValue  MaxValue=MaxValue  TriggerInit=[20 25 190 75]  MaskValue=MaskValue
      settings: SourceProductName=Bose Talaria
  wires:
  Tune Variable/1 -> TrivialTranslation/1  "MaxSpl"
  TrivialTranslation/1 -> TOP/1

== system Model_TranslationEngine64/NEAR/Near1p1/VolumeMute/VolMuteCh1/Ann1NonEntVncApplied/nonentVNCApplied_subsystem/TuneTOP ==
  Captured Tune Const : CapturedConstLib/CapturedConst  TriggerInit=[120 32 220 68]  Role=Automatic
      settings: SourceProductName=Bose Talaria
  Captured Tune Const1 : CapturedConstLib/CapturedConst  TriggerInit=[120 77 220 113]  Role=Automatic
      settings: SourceProductName=Bose Talaria
  TranslateTrigger : TuneVar/TranslateTrigger  TriggerInit=[306 -100 344 -45]
      settings: SourceProductName=Bose Talaria
  Translation : MATLAB Function  TreatAsAtomicUnit=on
  den : TOP/TOP  TriggerInit=[450 90 595 150]  TopName=den  DataTypeOut=single  BankNumber=0  PreOverlay=false  PostOverlay=false  Role=Automatic
      settings: SourceProductName=Bose Talaria
  num : TOP/TOP  TriggerInit=[450 -45 595 15]  TopName=Num  DataTypeOut=single  BankNumber=0  PreOverlay=false  PostOverlay=false  Role=Automatic
      settings: SourceProductName=Bose Talaria
  tuneVARTau : TuneVar/TuneVar  TuneName=Tau  SpecifyMaxSize=on  VariableDim=1 (Row)  MaxSize=[1 1]  TunabilityNumber=1  MinValue=[]  MaxValue=[]  TriggerInit=[-30 -85 140 -35]  MaskValue=Config.DefaultTau
      settings: SourceProductName=Bose Talaria
  wires:
  Captured Tune Const1/1 -> Translation/3(L)
  Captured Tune Const/1 -> Translation/2(Fs)
  Translation/2(Den) -> den/1
  Translation/1(Num) -> num/1
  tuneVARTau/1 -> Translation/1(tau)  "Tau"
  TranslateTrigger/1 -> Translation/Trigger

== system Model_TranslationEngine64/NEAR/Near1p1/VolumeMute/VolMuteCh1/Mute/MuteControl/TuneVarRampTime ==
  TOP : TOP/TOP  TriggerInit=[440 20 585 80]  TopName=RampTime  DataTypeOut=single  BankNumber=BankNumber  PreOverlay=PreOverlay  PostOverlay=PostOverlay  Role=Automatic
      settings: SourceProductName=Bose Talaria
  TrivialTranslation : TuneVar/TrivialTranslation  TriggerInit=[300 28 350 72]
      settings: SourceProductName=Bose Talaria
  Tune Variable : TuneVar/TuneVar  TuneName=RampTime  SpecifyMaxSize=off  VariableDim=1 (Row)  MaxSize=[1 1]  TunabilityNumber=1  MinValue=MinValue  MaxValue=MaxValue  TriggerInit=[20 25 190 75]  MaskValue=MaskValue
      settings: SourceProductName=Bose Talaria
  wires:
  Tune Variable/1 -> TrivialTranslation/1  "RampTime"
  TrivialTranslation/1 -> TOP/1

== system Model_TranslationEngine64/NEAR/Near1p1/VolumeMute/VolMuteCh2/Ann2NonEntGainCalc/vncSignal/TuneTOP ==
  TOP : TOP/TOP  TriggerInit=[440 20 585 80]  TopName=MinVncSignal  DataTypeOut=single  BankNumber=BankNumber  PreOverlay=PreOverlay  PostOverlay=PostOverlay  Role=Automatic
      settings: SourceProductName=Bose Talaria
  TrivialTranslation : TuneVar/TrivialTranslation  TriggerInit=[300 28 350 72]
      settings: SourceProductName=Bose Talaria
  Tune Variable : TuneVar/TuneVar  TuneName=MinVncSignal  SpecifyMaxSize=off  VariableDim=1 (Row)  MaxSize=[1 1]  TunabilityNumber=1  MinValue=MinValue  MaxValue=MaxValue  TriggerInit=[20 25 190 75]  MaskValue=MaskValue
      settings: SourceProductName=Bose Talaria
  wires:
  Tune Variable/1 -> TrivialTranslation/1  "MinVncSignal"
  TrivialTranslation/1 -> TOP/1

== system Model_TranslationEngine64/NEAR/Near1p1/VolumeMute/VolMuteCh2/Ann2NonEntGainCalc/vncSignal/TuneTOP1 ==
  TOP : TOP/TOP  TriggerInit=[440 20 585 80]  TopName=MaxSpl  DataTypeOut=single  BankNumber=BankNumber  PreOverlay=PreOverlay  PostOverlay=PostOverlay  Role=Automatic
      settings: SourceProductName=Bose Talaria
  TrivialTranslation : TuneVar/TrivialTranslation  TriggerInit=[300 28 350 72]
      settings: SourceProductName=Bose Talaria
  Tune Variable : TuneVar/TuneVar  TuneName=MaxSpl  SpecifyMaxSize=off  VariableDim=1 (Row)  MaxSize=[1 1]  TunabilityNumber=1  MinValue=MinValue  MaxValue=MaxValue  TriggerInit=[20 25 190 75]  MaskValue=MaskValue
      settings: SourceProductName=Bose Talaria
  wires:
  Tune Variable/1 -> TrivialTranslation/1  "MaxSpl"
  TrivialTranslation/1 -> TOP/1

== system Model_TranslationEngine64/NEAR/Near1p1/VolumeMute/VolMuteCh2/Ann2NonEntVncApplied/nonentVNCApplied_subsystem/TuneTOP ==
  Captured Tune Const : CapturedConstLib/CapturedConst  TriggerInit=[120 32 220 68]  Role=Automatic
      settings: SourceProductName=Bose Talaria
  Captured Tune Const1 : CapturedConstLib/CapturedConst  TriggerInit=[120 77 220 113]  Role=Automatic
      settings: SourceProductName=Bose Talaria
  TranslateTrigger : TuneVar/TranslateTrigger  TriggerInit=[306 -100 344 -45]
      settings: SourceProductName=Bose Talaria
  Translation : MATLAB Function  TreatAsAtomicUnit=on
  den : TOP/TOP  TriggerInit=[450 90 595 150]  TopName=den  DataTypeOut=single  BankNumber=0  PreOverlay=false  PostOverlay=false  Role=Automatic
      settings: SourceProductName=Bose Talaria
  num : TOP/TOP  TriggerInit=[450 -45 595 15]  TopName=Num  DataTypeOut=single  BankNumber=0  PreOverlay=false  PostOverlay=false  Role=Automatic
      settings: SourceProductName=Bose Talaria
  tuneVARTau : TuneVar/TuneVar  TuneName=Tau  SpecifyMaxSize=on  VariableDim=1 (Row)  MaxSize=[1 1]  TunabilityNumber=1  MinValue=[]  MaxValue=[]  TriggerInit=[-30 -85 140 -35]  MaskValue=Config.DefaultTau
      settings: SourceProductName=Bose Talaria
  wires:
  Captured Tune Const1/1 -> Translation/3(L)
  Captured Tune Const/1 -> Translation/2(Fs)
  Translation/2(Den) -> den/1
  Translation/1(Num) -> num/1
  tuneVARTau/1 -> Translation/1(tau)  "Tau"
  TranslateTrigger/1 -> Translation/Trigger

== system Model_TranslationEngine64/NEAR/Near1p1/VolumeMute/VolMuteCh2/Mute/MuteControl/TuneVarRampTime ==
  TOP : TOP/TOP  TriggerInit=[440 20 585 80]  TopName=RampTime  DataTypeOut=single  BankNumber=BankNumber  PreOverlay=PreOverlay  PostOverlay=PostOverlay  Role=Automatic
      settings: SourceProductName=Bose Talaria
  TrivialTranslation : TuneVar/TrivialTranslation  TriggerInit=[300 28 350 72]
      settings: SourceProductName=Bose Talaria
  Tune Variable : TuneVar/TuneVar  TuneName=RampTime  SpecifyMaxSize=off  VariableDim=1 (Row)  MaxSize=[1 1]  TunabilityNumber=1  MinValue=MinValue  MaxValue=MaxValue  TriggerInit=[20 25 190 75]  MaskValue=MaskValue
      settings: SourceProductName=Bose Talaria
  wires:
  Tune Variable/1 -> TrivialTranslation/1  "RampTime"
  TrivialTranslation/1 -> TOP/1

== system Model_TranslationEngine64/NEAR/Near1p1/VolumeMute/VolMuteCh3/Ann3NonEntGainCalc/vncSignal/TuneTOP ==
  TOP : TOP/TOP  TriggerInit=[440 20 585 80]  TopName=MinVncSignal  DataTypeOut=single  BankNumber=BankNumber  PreOverlay=PreOverlay  PostOverlay=PostOverlay  Role=Automatic
      settings: SourceProductName=Bose Talaria
  TrivialTranslation : TuneVar/TrivialTranslation  TriggerInit=[300 28 350 72]
      settings: SourceProductName=Bose Talaria
  Tune Variable : TuneVar/TuneVar  TuneName=MinVncSignal  SpecifyMaxSize=off  VariableDim=1 (Row)  MaxSize=[1 1]  TunabilityNumber=1  MinValue=MinValue  MaxValue=MaxValue  TriggerInit=[20 25 190 75]  MaskValue=MaskValue
      settings: SourceProductName=Bose Talaria
  wires:
  Tune Variable/1 -> TrivialTranslation/1  "MinVncSignal"
  TrivialTranslation/1 -> TOP/1

== system Model_TranslationEngine64/NEAR/Near1p1/VolumeMute/VolMuteCh3/Ann3NonEntGainCalc/vncSignal/TuneTOP1 ==
  TOP : TOP/TOP  TriggerInit=[440 20 585 80]  TopName=MaxSpl  DataTypeOut=single  BankNumber=BankNumber  PreOverlay=PreOverlay  PostOverlay=PostOverlay  Role=Automatic
      settings: SourceProductName=Bose Talaria
  TrivialTranslation : TuneVar/TrivialTranslation  TriggerInit=[300 28 350 72]
      settings: SourceProductName=Bose Talaria
  Tune Variable : TuneVar/TuneVar  TuneName=MaxSpl  SpecifyMaxSize=off  VariableDim=1 (Row)  MaxSize=[1 1]  TunabilityNumber=1  MinValue=MinValue  MaxValue=MaxValue  TriggerInit=[20 25 190 75]  MaskValue=MaskValue
      settings: SourceProductName=Bose Talaria
  wires:
  Tune Variable/1 -> TrivialTranslation/1  "MaxSpl"
  TrivialTranslation/1 -> TOP/1

== system Model_TranslationEngine64/NEAR/Near1p1/VolumeMute/VolMuteCh3/Ann3NonEntVncApplied/nonentVNCApplied_subsystem/TuneTOP ==
  Captured Tune Const : CapturedConstLib/CapturedConst  TriggerInit=[120 32 220 68]  Role=Automatic
      settings: SourceProductName=Bose Talaria
  Captured Tune Const1 : CapturedConstLib/CapturedConst  TriggerInit=[120 77 220 113]  Role=Automatic
      settings: SourceProductName=Bose Talaria
  TranslateTrigger : TuneVar/TranslateTrigger  TriggerInit=[306 -100 344 -45]
      settings: SourceProductName=Bose Talaria
  Translation : MATLAB Function  TreatAsAtomicUnit=on
  den : TOP/TOP  TriggerInit=[450 90 595 150]  TopName=den  DataTypeOut=single  BankNumber=0  PreOverlay=false  PostOverlay=false  Role=Automatic
      settings: SourceProductName=Bose Talaria
  num : TOP/TOP  TriggerInit=[450 -45 595 15]  TopName=Num  DataTypeOut=single  BankNumber=0  PreOverlay=false  PostOverlay=false  Role=Automatic
      settings: SourceProductName=Bose Talaria
  tuneVARTau : TuneVar/TuneVar  TuneName=Tau  SpecifyMaxSize=on  VariableDim=1 (Row)  MaxSize=[1 1]  TunabilityNumber=1  MinValue=[]  MaxValue=[]  TriggerInit=[-30 -85 140 -35]  MaskValue=Config.DefaultTau
      settings: SourceProductName=Bose Talaria
  wires:
  Captured Tune Const1/1 -> Translation/3(L)
  Captured Tune Const/1 -> Translation/2(Fs)
  Translation/2(Den) -> den/1
  Translation/1(Num) -> num/1
  tuneVARTau/1 -> Translation/1(tau)  "Tau"
  TranslateTrigger/1 -> Translation/Trigger

== system Model_TranslationEngine64/NEAR/Near1p1/VolumeMute/VolMuteCh3/Mute/MuteControl/TuneVarRampTime ==
  TOP : TOP/TOP  TriggerInit=[440 20 585 80]  TopName=RampTime  DataTypeOut=single  BankNumber=BankNumber  PreOverlay=PreOverlay  PostOverlay=PostOverlay  Role=Automatic
      settings: SourceProductName=Bose Talaria
  TrivialTranslation : TuneVar/TrivialTranslation  TriggerInit=[300 28 350 72]
      settings: SourceProductName=Bose Talaria
  Tune Variable : TuneVar/TuneVar  TuneName=RampTime  SpecifyMaxSize=off  VariableDim=1 (Row)  MaxSize=[1 1]  TunabilityNumber=1  MinValue=MinValue  MaxValue=MaxValue  TriggerInit=[20 25 190 75]  MaskValue=MaskValue
      settings: SourceProductName=Bose Talaria
  wires:
  Tune Variable/1 -> TrivialTranslation/1  "RampTime"
  TrivialTranslation/1 -> TOP/1

== system Model_TranslationEngine64/NEAR/Near1p1/VolumeMute/VolMuteCh4/Ann4NonEntGainCalc/vncSignal/TuneTOP ==
  TOP : TOP/TOP  TriggerInit=[440 20 585 80]  TopName=MinVncSignal  DataTypeOut=single  BankNumber=BankNumber  PreOverlay=PreOverlay  PostOverlay=PostOverlay  Role=Automatic
      settings: SourceProductName=Bose Talaria
  TrivialTranslation : TuneVar/TrivialTranslation  TriggerInit=[300 28 350 72]
      settings: SourceProductName=Bose Talaria
  Tune Variable : TuneVar/TuneVar  TuneName=MinVncSignal  SpecifyMaxSize=off  VariableDim=1 (Row)  MaxSize=[1 1]  TunabilityNumber=1  MinValue=MinValue  MaxValue=MaxValue  TriggerInit=[20 25 190 75]  MaskValue=MaskValue
      settings: SourceProductName=Bose Talaria
  wires:
  Tune Variable/1 -> TrivialTranslation/1  "MinVncSignal"
  TrivialTranslation/1 -> TOP/1

== system Model_TranslationEngine64/NEAR/Near1p1/VolumeMute/VolMuteCh4/Ann4NonEntGainCalc/vncSignal/TuneTOP1 ==
  TOP : TOP/TOP  TriggerInit=[440 20 585 80]  TopName=MaxSpl  DataTypeOut=single  BankNumber=BankNumber  PreOverlay=PreOverlay  PostOverlay=PostOverlay  Role=Automatic
      settings: SourceProductName=Bose Talaria
  TrivialTranslation : TuneVar/TrivialTranslation  TriggerInit=[300 28 350 72]
      settings: SourceProductName=Bose Talaria
  Tune Variable : TuneVar/TuneVar  TuneName=MaxSpl  SpecifyMaxSize=off  VariableDim=1 (Row)  MaxSize=[1 1]  TunabilityNumber=1  MinValue=MinValue  MaxValue=MaxValue  TriggerInit=[20 25 190 75]  MaskValue=MaskValue
      settings: SourceProductName=Bose Talaria
  wires:
  Tune Variable/1 -> TrivialTranslation/1  "MaxSpl"
  TrivialTranslation/1 -> TOP/1

== system Model_TranslationEngine64/NEAR/Near1p1/VolumeMute/VolMuteCh4/Ann4NonEntVncApplied/nonentVNCApplied_subsystem/TuneTOP ==
  Captured Tune Const : CapturedConstLib/CapturedConst  TriggerInit=[120 32 220 68]  Role=Automatic
      settings: SourceProductName=Bose Talaria
  Captured Tune Const1 : CapturedConstLib/CapturedConst  TriggerInit=[120 77 220 113]  Role=Automatic
      settings: SourceProductName=Bose Talaria
  TranslateTrigger : TuneVar/TranslateTrigger  TriggerInit=[306 -100 344 -45]
      settings: SourceProductName=Bose Talaria
  Translation : MATLAB Function  TreatAsAtomicUnit=on
  den : TOP/TOP  TriggerInit=[450 90 595 150]  TopName=den  DataTypeOut=single  BankNumber=0  PreOverlay=false  PostOverlay=false  Role=Automatic
      settings: SourceProductName=Bose Talaria
  num : TOP/TOP  TriggerInit=[450 -45 595 15]  TopName=Num  DataTypeOut=single  BankNumber=0  PreOverlay=false  PostOverlay=false  Role=Automatic
      settings: SourceProductName=Bose Talaria
  tuneVARTau : TuneVar/TuneVar  TuneName=Tau  SpecifyMaxSize=on  VariableDim=1 (Row)  MaxSize=[1 1]  TunabilityNumber=1  MinValue=[]  MaxValue=[]  TriggerInit=[-30 -85 140 -35]  MaskValue=Config.DefaultTau
      settings: SourceProductName=Bose Talaria
  wires:
  Captured Tune Const1/1 -> Translation/3(L)
  Captured Tune Const/1 -> Translation/2(Fs)
  Translation/2(Den) -> den/1
  Translation/1(Num) -> num/1
  tuneVARTau/1 -> Translation/1(tau)  "Tau"
  TranslateTrigger/1 -> Translation/Trigger

== system Model_TranslationEngine64/NEAR/Near1p1/VolumeMute/VolMuteCh4/Mute/MuteControl/TuneVarRampTime ==
  TOP : TOP/TOP  TriggerInit=[440 20 585 80]  TopName=RampTime  DataTypeOut=single  BankNumber=BankNumber  PreOverlay=PreOverlay  PostOverlay=PostOverlay  Role=Automatic
      settings: SourceProductName=Bose Talaria
  TrivialTranslation : TuneVar/TrivialTranslation  TriggerInit=[300 28 350 72]
      settings: SourceProductName=Bose Talaria
  Tune Variable : TuneVar/TuneVar  TuneName=RampTime  SpecifyMaxSize=off  VariableDim=1 (Row)  MaxSize=[1 1]  TunabilityNumber=1  MinValue=MinValue  MaxValue=MaxValue  TriggerInit=[20 25 190 75]  MaskValue=MaskValue
      settings: SourceProductName=Bose Talaria
  wires:
  Tune Variable/1 -> TrivialTranslation/1  "RampTime"
  TrivialTranslation/1 -> TOP/1

== system Model_TranslationEngine64/ModelPreAmp/DecRate/AudioPilot35/Audiopilot_3_5/GainApplication/Compensation/MidrangeLpfAlignDelay/AlignDelay ==
  Captured Tune Const : CapturedConstLib/CapturedConst  TriggerInit=[255 62 355 98]  Role=Automatic
      settings: SourceProductName=Bose Talaria
  MaxCheck : MATLAB Function  TreatAsAtomicUnit=on
  TOP : TOP/TOP  TriggerInit=[540 17 745 83]  TopName=MidrangeLpfAlignDelaySamples  DataTypeOut=int32  BankNumber=0  PreOverlay=false  PostOverlay=false  Role=Automatic
      settings: SourceProductName=Bose Talaria
  TranslateTrigger : TuneVar/TranslateTrigger  TriggerInit=[446 -125 484 -70]
      settings: SourceProductName=Bose Talaria
  Tune Variable : TuneVar/TuneVar  TuneName=MidrangeLpfAlignDelaySamples  SpecifyMaxSize=off  VariableDim=1 (Row)  MaxSize=[1 1]  TunabilityNumber=1  MinValue=[]  MaxValue=[]  TriggerInit=[-50 -10 220 40]  MaskValue=Config.MidrangeLpfAlignDelaySamples
      settings: SourceProductName=Bose Talaria
  wires:
  Tune Variable/1 -> MaxCheck/1(DelaySamples)  "MidrangeLpfAlignDelaySamples"
  MaxCheck/1(Samples) -> TOP/1
  TranslateTrigger/1 -> MaxCheck/Trigger
  Captured Tune Const/1 -> MaxCheck/2(MaxDelaySamples)

== system Model_TranslationEngine64/ModelPreAmp/DecRate/AudioPilot35/Audiopilot_3_5/GainCalculation/Boosts/InputOverride/MinSignalLevel ==
  TOP : TOP/TOP  TriggerInit=[440 20 585 80]  TopName=MinSignalLevelDbspl  DataTypeOut=single  BankNumber=BankNumber  PreOverlay=PreOverlay  PostOverlay=PostOverlay  Role=Automatic
      settings: SourceProductName=Bose Talaria
  TrivialTranslation : TuneVar/TrivialTranslation  TriggerInit=[300 28 350 72]
      settings: SourceProductName=Bose Talaria
  Tune Variable : TuneVar/TuneVar  TuneName=MinSignalLevelDbspl  SpecifyMaxSize=off  VariableDim=1 (Row)  MaxSize=[1 1]  TunabilityNumber=1  MinValue=MinValue  MaxValue=MaxValue  TriggerInit=[20 25 190 75]  MaskValue=MaskValue
      settings: SourceProductName=Bose Talaria
  wires:
  TrivialTranslation/1 -> TOP/1
  Tune Variable/1 -> TrivialTranslation/1  "MinSignalLevelDbspl"
